simulink library "libwind"  (Simulink 7.9)
settings: Solver=ode45  StartTime=0.0  StopTime=10.0  RelTol=1e-3
libraries: simulink x2
settings Model: Creator=grunnet  LastModifiedBy=tom

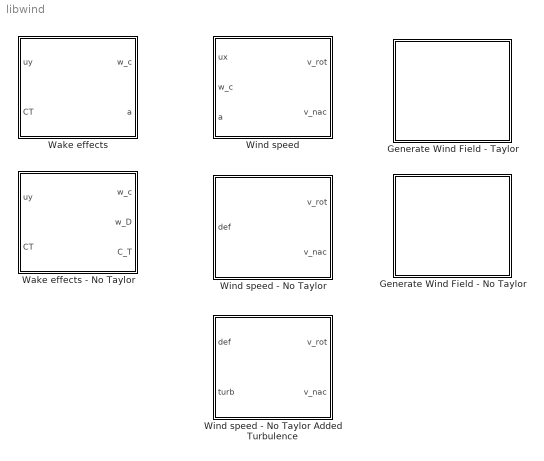
== system libwind ==
  Generate Wind Field - No Taylor : Subsystem
      settings: OpenFcn=create_windfield_no_taylor()
      mask Type: Wind field generation
      mask Description: Generates a wind field
      mask Display: image(imread('wind.jpg'))
  Generate Wind Field - Taylor : Subsystem
      settings: OpenFcn=create_windfield()
      mask Type: Wind field generation
      mask Description: Generates a wind field
      mask Display: image(imread('wind.jpg'))
  Wake effects : Subsystem  mask(Wind){}
      mask help: Calculates wake effects based on turbine CT and crosswinds
      mask init:
      | p=get_param(gcb,'UserData');
      mask Display:
      | image(imread('Wake.JPG'))
      | 
      | port_label('output',1,'WC [m]')
      | port_label('output',2,'a')
      | 
      | 
      | port_label('input',1,'U_y [m/s]')
      | port_label('input',2,'CT')
  Wake effects - No Taylor : Subsystem  mask(Wind){}
      mask help: Calculates wake effects based on turbine CT and crosswinds
      mask init:
      | p=get_param(gcb,'UserData');
      mask Display:
      | image(imread('Wake.JPG'))
      | 
      | port_label('output',1,'WC [m]')
      | port_label('output',2,'WD [m]')
      | port_label('output',3,'CT_dw')
      | 
      | 
      | port_label('input',1,'U_y [m/s]')
      | port_label('input',2,'CT')
  Wind speed : Subsystem  mask(Wind){}
      mask help: Calculates average over rotor and nacelle wind speeds based on wake effects
      mask init:
      | p=get_param(gcb,'UserData');
      mask Display:
      | image(imread('anemometer.jpg'))
      | 
      | port_label('output',1,'v_rot [m/s]')
      | port_label('output',2,'v_nac [m/s]')
      | 
      | 
      | port_label('input',1,'U_x [m/s]')
      | port_label('input',2,'WC [m]')
      | port_label('input',3,'a')
  Wind speed - No Taylor : Subsystem  mask(Wind){}
      mask help: Calculates average over rotor and nacelle wind speeds based on wake effects
      mask init:
      | p=get_param(gcb,'UserData');
      mask Display:
      | image(imread('anemometer.jpg'))
      | 
      | port_label('output',1,'v_rot [m/s]')
      | port_label('output',2,'v_nac [m/s]')
      | %port_label('output',3,'deficit')
      | 
      | %port_label('input',1,'U_x [m/s]')
      | %port_label('input',1,'WC [m]')
      | %port_label('input',2,'WD [m]')
      | %port_label('input',3,'CT_dw')
      | 
      | port_label('input',1,'deficit')
  Wind speed - No Taylor Added Turbulence : Subsystem  RequirementInfo="{}  %GIDa_19238d34_3b8b_4f4f_8e53_e60f202c3814"  mask(Wind){}
      mask help: Calculates average over rotor and nacelle wind speeds based on wake effects
      mask init:
      | p=get_param(gcb,'UserData');
      mask Display:
      | image(imread('anemometer.jpg'))
      | 
      | port_label('output',1,'v_rot [m/s]')
      | port_label('output',2,'v_nac [m/s]')
      | %port_label('output',3,'deficit')
      | 
      | %port_label('input',1,'U_x [m/s]')
      | %port_label('input',1,'WC [m]')
      | %port_label('input',2,'WD [m]')
      | %port_label('input',3,'CT_dw')
      | 
      | port_label('input',1,'deficit')

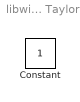
== system libwind/Generate Wind Field - No Taylor ==
  Constant : Constant

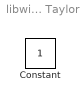
== system libwind/Generate Wind Field - Taylor ==
  Constant : Constant

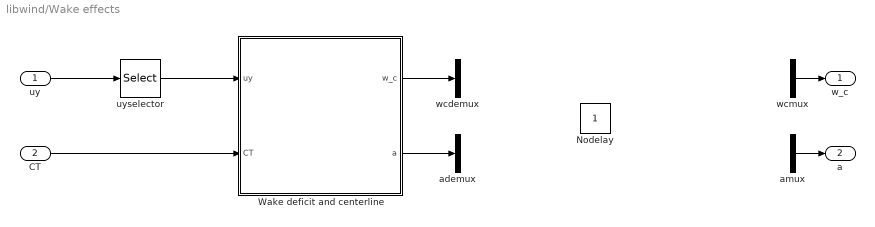
== system libwind/Wake effects ==
  uy : Inport
  CT : Inport  Port=2
  Nodelay : Constant
  Wake deficit and centerline : MATLAB Function  TreatAsAtomicUnit=on
  ademux : Demux  Outputs=2
  amux : Mux  Inputs=2
  uyselector : Selector  NumberOfDimensions=2  InputPortWidth=3  IndexOptions=Select all,Index vector (dialog)  Indices=[1 3],p.wt.num  OutputSizes=1,1
  wcdemux : Demux  Outputs=2
  wcmux : Mux  Inputs=2
  w_c : Outport
  a : Outport  Port=2
  wires:
  CT/1 -> Wake deficit and centerline/2(CT)
  uy/1 -> uyselector/1
  uyselector/1 -> Wake deficit and centerline/1(uy)
  Wake deficit and centerline/1(w_c) -> wcdemux/1
  Wake deficit and centerline/2(a) -> ademux/1
  wcmux/1 -> w_c/1
  amux/1 -> a/1

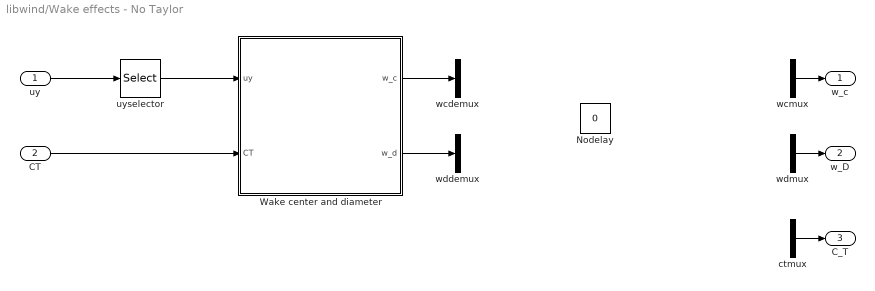
== system libwind/Wake effects - No Taylor ==
  uy : Inport
  CT : Inport  Port=2
  Nodelay : Constant  Value=0
  Wake center and diameter : MATLAB Function  TreatAsAtomicUnit=on
  ctmux : Mux  Inputs=2
  uyselector : Selector  NumberOfDimensions=2  InputPortWidth=3  IndexOptions=Select all,Index vector (dialog)  Indices=[1 3],p.wt.num  OutputSizes=1,1
  wcdemux : Demux  Outputs=2
  wcmux : Mux  Inputs=2
  wddemux : Demux  Outputs=2
  wdmux : Mux  Inputs=2
  w_c : Outport
  w_D : Outport  Port=2
  C_T : Outport  Port=3
  wires:
  wdmux/1 -> w_D/1
  wcmux/1 -> w_c/1
  Wake center and diameter/2(w_d) -> wddemux/1
  Wake center and diameter/1(w_c) -> wcdemux/1
  uyselector/1 -> Wake center and diameter/1(uy)
  uy/1 -> uyselector/1
  CT/1 -> Wake center and diameter/2(CT)
  ctmux/1 -> C_T/1

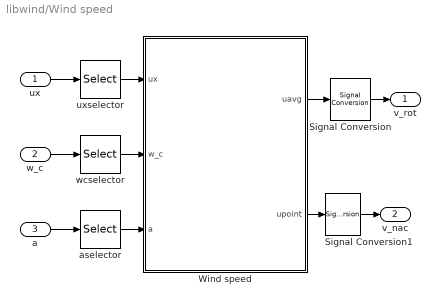
== system libwind/Wind speed ==
  ux : Inport
  w_c : Inport  Port=2
  a : Inport  Port=3
  Signal Conversion : SignalConversion  ConversionOutput=Contiguous copy
  Signal Conversion1 : SignalConversion  ConversionOutput=Contiguous copy
  Wind speed : MATLAB Function  TreatAsAtomicUnit=on
  aselector : Selector  NumberOfDimensions=2  InputPortWidth=3  IndexOptions=Index vector (dialog),Select all  Indices=p.wt.num,p.wt.num  OutputSizes=1,1
  uxselector : Selector  NumberOfDimensions=2  InputPortWidth=3  IndexOptions=Select all,Index vector (dialog)  Indices=[1 3],p.wt.num  OutputSizes=1,1
  wcselector : Selector  NumberOfDimensions=2  InputPortWidth=3  IndexOptions=Index vector (dialog),Select all  Indices=p.wt.num,p.wt.num  OutputSizes=1,1
  v_rot : Outport
  v_nac : Outport  Port=2
  wires:
  Wind speed/2(upoint) -> Signal Conversion1/1
  Wind speed/1(uavg) -> Signal Conversion/1
  ux/1 -> uxselector/1
  w_c/1 -> wcselector/1
  wcselector/1 -> Wind speed/2(w_c)
  a/1 -> aselector/1
  aselector/1 -> Wind speed/3(a)
  uxselector/1 -> Wind speed/1(ux)
  Signal Conversion/1 -> v_rot/1
  Signal Conversion1/1 -> v_nac/1

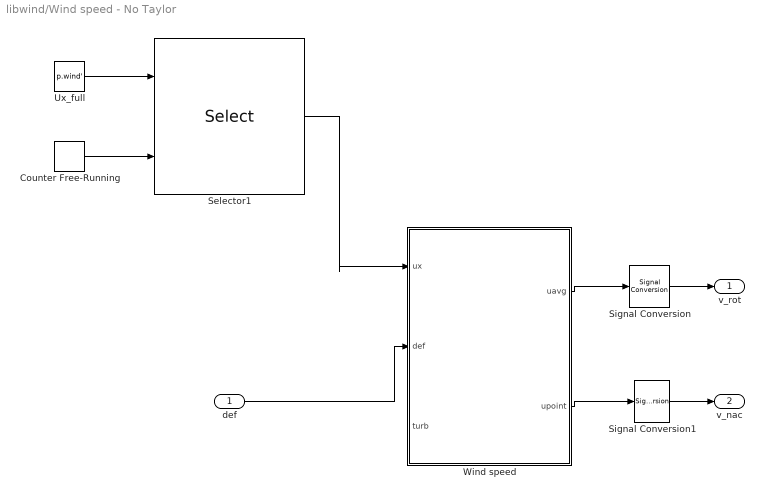
== system libwind/Wind speed - No Taylor ==
  def : Inport
  Counter Free-Running : simulink/Sources/Counter Free-Running  NumBits=32  tsamp=p.ts
  Selector1 : Selector  NumberOfDimensions=2  IndexMode=Zero-based  InputPortWidth=3  IndexOptions=Select all,Index vector (port)  Indices=[1 3],1  OutputSizes=1,1
  Signal Conversion : SignalConversion  ConversionOutput=Contiguous copy
  Signal Conversion1 : SignalConversion  ConversionOutput=Contiguous copy
  Ux_full : Constant  Value=p.wind'
  Wind speed : MATLAB Function  TreatAsAtomicUnit=on
  v_rot : Outport
  v_nac : Outport  Port=2
  wires:
  Signal Conversion1/1 -> v_nac/1
  Signal Conversion/1 -> v_rot/1
  Selector1/1 -> Wind speed/1(ux)
  Ux_full/1 -> Selector1/1
  Counter Free-Running/1 -> Selector1/2
  Wind speed/1(uavg) -> Signal Conversion/1
  Wind speed/2(upoint) -> Signal Conversion1/1
  def/1 -> Wind speed/2(def)

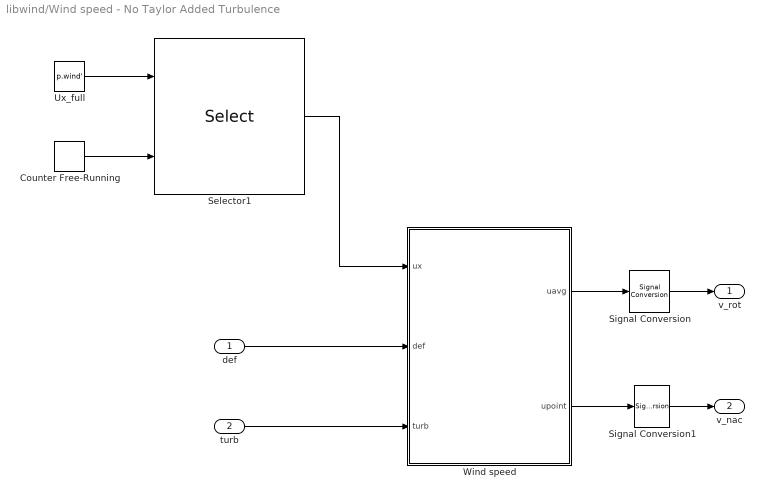
== system libwind/Wind speed - No Taylor Added Turbulence ==
  def : Inport  RequirementInfo="{}  %GIDa_854ad8b6_da7d_4249_9f90_7e96f7ebbea5"
  turb : Inport  RequirementInfo="{}  %GIDa_c86b1add_b9b9_44e5_b162_6ac8e6c91ac6"  Port=2
  Counter Free-Running : simulink/Sources/Counter Free-Running  NumBits=32  tsamp=p.ts
  Selector1 : Selector  NumberOfDimensions=2  IndexMode=Zero-based  InputPortWidth=3  IndexOptions=Select all,Index vector (port)  Indices=[1 3],1  OutputSizes=1,1
  Signal Conversion : SignalConversion  ConversionOutput=Contiguous copy
  Signal Conversion1 : SignalConversion  ConversionOutput=Contiguous copy
  Ux_full : Constant  Value=p.wind'
  Wind speed : MATLAB Function  TreatAsAtomicUnit=on
  v_rot : Outport
  v_nac : Outport  Port=2
  wires:
  def/1 -> Wind speed/2(def)
  Wind speed/2(upoint) -> Signal Conversion1/1
  Wind speed/1(uavg) -> Signal Conversion/1
  Counter Free-Running/1 -> Selector1/2
  Ux_full/1 -> Selector1/1
  Selector1/1 -> Wind speed/1(ux)
  Signal Conversion/1 -> v_rot/1
  Signal Conversion1/1 -> v_nac/1
  turb/1 -> Wind speed/3(turb)

== matlab function Wake effects - No Taylor/Wake center and diameter ==
  data: uy input double; CT input double; p parameter double; w_c output double; w_d output double
function [w_c,w_d]=wake(uy,CT,p)
    % Todo: Change length(uy)*grid_size to farm size?
    %       Change such that parm is passed directly

    w_c=zeros(length(p.farm.x),1);
    w_d=zeros(length(p.farm.x),1);
    if CT < 1
        beta_w = (1+sqrt(1-CT))/(2*sqrt(1-CT));
    else
        beta_w = 1;
    end
    %beta_w = (1+sqrt(1-CT))/(2*sqrt(1-CT));
    %Find wake center and deficit for all other turbines
    for i=1:length(p.farm.x)
        delta_dist = p.farm.x(i)-p.wt.x;
        if(delta_dist>0) %Is turbine P downwind?
            w_d(i)= (beta_w^(p.k/2) +p.alpha*delta_dist/(2*p.wt.rotor.r))^(1/p.k)*2*p.wt.rotor.r;
            w_c(i)=wakecenter(uy,p.farm.x(i),p);%max(min(wakecenter(uy,p.farm.x(i),p),p.grid.ysize),1);
            
        else
            w_c(i)=p.wt.y;
            w_d(i)=0;
        end
    end
end


function wc=wakecenter(uy,px,p)
    
    %computer number of grid points to px
    it=ceil((px-p.wt.x)/p.grid.size);
    
    wc=p.wt.y; %wake center starts at turbine position
    
    for i=1:it %Compute the meandering for each grid point
        uysum=0;
        %compute the grid number for low meandering edge
        m_min=max(floor((wc-p.wt.meand.r(i))/p.grid.size)+1,1); 
        %compute the grid number for the high meandering edge
        m_max=min(ceil((wc+p.wt.meand.r(i))/p.grid.size)+1,length(uy)); 
        
        %average transversal velocity over the wake area
        for j=m_min:m_max
            uysum=uysum+uy(j);
        end
        uyavg=uysum/(m_max-m_min+1);
        
        % wake center filtered
        % Should be calculated from mean air speed vs uyavg and lowpass filtered
        % Redo filter computation
        % yeff=ts*uyavg=grid.size/uxmean*uyavg
        % wc=wc+alpha*uyavg
        
        %Uncomment to reproduce bug
        %wc=p.wt.y;
        
        %Uncomment to reproduce meandering limits
        %wc=min(max(wc,p.wt.y-150),p.wt.y+150);
        
        %Notice here ts such that wake moves with uyavg speed
        wc=wc+p.ts*uyavg;
    end
end

== matlab function Wind speed - No Taylor/Wind speed ==
  data: ux input double; def input double; turb input double; p parameter double; uavg output double; upoint output double
function [uavg, upoint] = windspeed(ux,def,turb,p) %#eml
% ux    is the wind vector at the x position of the turbine
% def   is the vector deficits at each turbine
% p     is a structure containing parameters  

%old deficit calculations w.o. added turbulence
%uavg = def(p.wt.num)*sum(ux)/(p.wind_grid);
%upoint = def(p.wt.num)*ux(ceil(p.wind_grid/2));

%the following is probably wrong
ux = sqrt(turb(p.wt.num))*(ux - p.U0) + p.U0; 
uavg = def(p.wt.num)*sum(ux)/(p.wind_grid);
upoint = def(p.wt.num)*ux(ceil(p.wind_grid/2));


%the following is probably correct
%ux = sqrt(turb(p.wt.num))*(ux - p.U0) + def(p.wt.num)*p.U0; 
%uavg = sum(ux)/(p.wind_grid);
%upoint = ux(ceil(p.wind_grid/2));

== matlab function Wake effects/Wake deficit and centerline ==
  data: uy input double; CT input double; p parameter double; w_c output double; a output double
function [w_c,a]=wake(uy,CT,p)
    % Todo: Change length(uy)*grid_size to farm size?
    %       Change such that parm is passed directly

    w_c=zeros(length(p.farm.x),1);
    a=ones(length(p.farm.x),1);
    
    %Find wake center and deficit for all other turbines
    for i=1:length(p.farm.x)
        if(p.farm.x(i)-p.wt.x>0) %Is turbine P downwind?
            w_c(i)=max(min(wakecenter(uy,p.farm.x(i),p),p.grid.ysize),1);
            a(i)=deficit(CT,p.farm.x(i),p);
        else
            w_c(i)=p.wt.y;
            a(i)=1;
        end
    end
end


function wc=wakecenter(uy,px,p)
    
    %computer number of grid points to px
    it=ceil((px-p.wt.x)/p.grid.size);
    
    wc=p.wt.y; %wake center starts at turbine position
    
    for i=1:it %Compute the meandering for each grid point
        uysum=0;
        %compute the grid number for low meandering edge
        m_min=max(floor((wc-p.wt.meand.r(i))/p.grid.size)+1,1); 
        %compute the grid number for the high meandering edge
        m_max=min(ceil((wc+p.wt.meand.r(i))/p.grid.size)+1,length(uy)); 
        
        %average transversal velocity over the wake area
        for j=m_min:m_max
            uysum=uysum+uy(j);
        end
        uyavg=uysum/(m_max-m_min+1);
        
        % wake center filtered
        % Should be calculated from mean air speed vs uyavg and lowpass filtered
        % Redo filter computation
        % yeff=ts*uyavg=grid.size/uxmean*uyavg
        % wc=wc+alpha*uyavg
        
        %Uncomment to reproduce bug
        %wc=p.wt.y;
        
        %Uncomment to reproduce meandering limits
        %wc=min(max(wc,p.wt.y-150),p.wt.y+150);
        
        %Notice here ts such that wake moves with uyavg speed
        wc=wc+p.ts*uyavg;
    end
end

function a=deficit(CT,px,p)
    %wake deficit at px-wtx distance from turbine
    a=1-.5*CT/(1+(px-p.wt.x)/(4*p.wt.rotor.r));
end

== matlab function Wind speed/Wind speed ==
  data: ux input double; w_c input double; a input double; p parameter double; uavg output double; upoint output double
function [uavg,upoint]=windspeed(ux,w_c,a,p)
% ux    is the wind vector at the x position of the turbine
% w_c   is the vector of wake centers from the other turbins at the x position of the turbine
% a     is the vector of velocity deficits at this turbine from the other turbines
% P     is a structure containing parameters  
   
%Initialise variables
uxsum=0;
av=ones(p.grid.ysize,1);

%Merge the wake from all turbines upwind
for i=1:length(p.farm.x)
    if(p.farm.x(i)<p.wt.x) %only compute deficit effect from upstream turbines

        %compute the grid number for low meandering edge
        mn=floor((w_c(i)-p.wt.exprad(i))/p.grid.size)+1;
        m_min=max(mn,1); 
        %compute the grid number for the high meandering edge
        mx=floor((w_c(i)+p.wt.exprad(i))/p.grid.size)+1;
        m_max=min(mx,floor(p.grid.ysize/p.grid.size)+1);

        %Merge wakes
        for j=m_min:m_max
            av(j)=av(j)*a(i);
        end
    end
end
    


%Rotor grid points - Todo move to farm setup
%compute the grid number for low rotor edge
r_min=floor((p.wt.y-p.wt.rotor.r)/p.grid.size)+1; 
%compute the grid number for the high rotor edge
r_max=floor((p.wt.y+p.wt.rotor.r)/p.grid.size)+1;

%Sum the wake corrected x-velocities over the rotor dish area
for i=r_min:r_max
    uxsum=uxsum+ux(i)*av(i);
end

%Compute the average
uavg=uxsum/(r_max-r_min+1);

%Extract the wake corrected velocity at the nacelle
upoint=ux(floor(p.wt.y/p.grid.size)+1)*av(floor(p.wt.y/p.grid.size)+1);
    
end

== matlab function Wind speed - No Taylor Added Turbulence/Wind speed ==
  data: ux input double; def input double; turb input double; p parameter double; uavg output double; upoint output double
function [uavg, upoint] = windspeed(ux,def,turb,p) %#eml
% ux    is the wind vector at the x position of the turbine
% def   is the vector deficits at each turbine
% p     is a structure containing parameters  

%old deficit calculations w.o. added turbulence
%uavg = def(p.wt.num)*sum(ux)/(p.wind_grid);
%upoint = def(p.wt.num)*ux(ceil(p.wind_grid/2));

%the following is probably wrong
ux = turb(p.wt.num)*(ux - p.U0) + p.U0; 
uavg = def(p.wt.num)*sum(ux)/(p.wind_grid);
upoint = def(p.wt.num)*ux(ceil(p.wind_grid/2));


%the following is probably correct
%ux = turb(p.wt.num)*(ux - p.U0) + def(p.wt.num)*p.U0; 
%uavg = sum(ux)/(p.wind_grid);
%upoint = ux(ceil(p.wind_grid/2));
